simulink model "sampleModel1745"  (R2023a)
settings: Solver=VariableStepAuto  StartTime=0.0  StopTime=10.0  RelTol=1e-3
libraries: hdlsllib x3, simulink x2
settings Model: Creator=user1  LastModifiedBy=user1

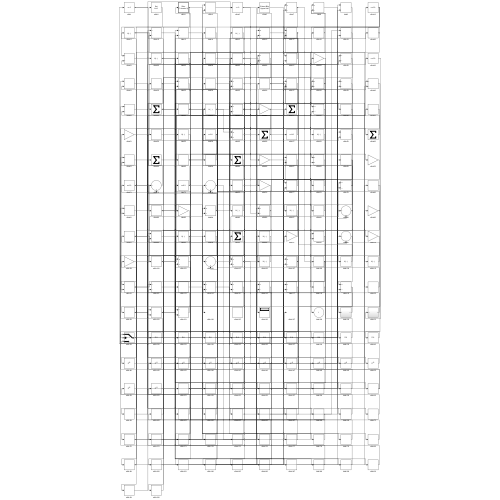
[thumbnail: Simulink's stored preview of the top-level diagram]
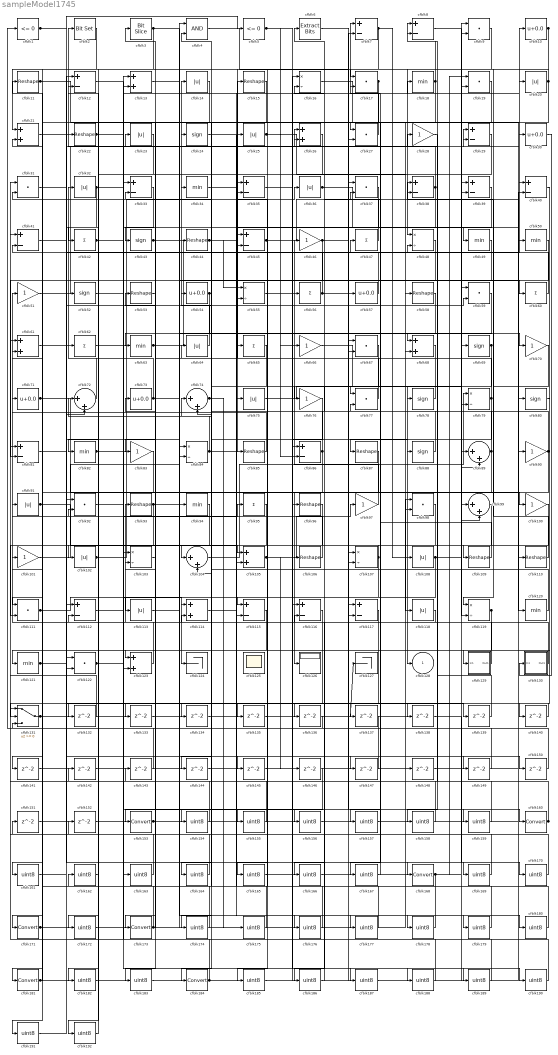
== system sampleModel1745 ==
  cfblk1 : hdlsllib/Logic and Bit Operations/Compare To Zero  relop=<=  OutDataTypeStr=boolean
  cfblk{10,30,54,57,71,73} (6 alike) : Bias  Bias=0.0  SaturateOnIntegerOverflow=off
  cfblk{28,46,51,66,70,76,83,90,97,100..101} (11 alike) : Gain
  cfblk{14,20,23,25,32,36,64,75,91,102,108,113,118} (13 alike) : Abs  SaturateOnIntegerOverflow=off
  cfblk{16,48,55,79,84,103,107,119} (8 alike) : Product  Inputs=*/  RndMeth=Zero  SaturateOnIntegerOverflow=on
  cfblk{72,74,89,99,104} (5 alike) : Sum  Inputs=|++
  cfblk{13,21,26,61,68,105,114,123} (8 alike) : Sum
  cfblk{11,15,22,44,53,58,85,87,93,96,106,109..110} (13 alike) : Reshape
  cfblk{9,17,19,27,31,37,59,67,77,92,98,111,122} (13 alike) : DotProduct  OutDataTypeStr=Inherit: Inherit via internal rule
  cfblk{7..8,12,29,33,35,38..41,45,81,86,112,115..117} (17 alike) : Sum  Inputs=+-
  cfblk{18,34,49..50,63,82,94,120..121} (9 alike) : MinMax
  cfblk124 : Terminator
  cfblk125 : Scope
      settings: Floating=on
  cfblk126 : Display
  cfblk127 : Terminator
  cfblk129 : Subsystem
      settings: LibrarySourceBlock=|
      | hdlsllib/Ports &
      | Subsystems/Subsystem
  cfblk130 : Subsystem
      settings: LibrarySourceBlock=|
      | hdlsllib/Ports &
      | Subsystems/Subsystem
  cfblk131 : Switch  SaturateOnIntegerOverflow=off  InputSameDT=off
  cfblk{132..152} (21 alike) : Delay  SampleTime=1
  cfblk{153,160,168,171,173,181,184} (7 alike) : DataTypeConversion  SaturateOnIntegerOverflow=off  RndMeth=Floor
  cfblk{154..159,161..167,169..170,172,174..180,182..183,185..192} (33 alike) : DataTypeConversion  OutDataTypeStr=uint8  SaturateOnIntegerOverflow=off  RndMeth=Floor
  cfblk2 : simulink/Logic and Bit Operations/Bit Set  iBit=0
      settings: LibrarySourceBlock=|
      | hdlsllib/Logic and Bit
      | Operations/Bit Set
  cfblk{24,43,52,69,78,80,88} (7 alike) : Signum
  cfblk3 : hdlsllib/Logic and Bit Operations/Bit Slice  lidx=7  ridx=0
  cfblk4 : Logic  AllPortsSameDT=off  OutDataTypeStr=boolean
  cfblk{42,47,56,60,62,65,95} (7 alike) : Sum  Inputs=+
  cfblk5 : hdlsllib/Logic and Bit Operations/Compare To Zero  relop=<=  OutDataTypeStr=boolean
  cfblk6 : simulink/Logic and Bit Operations/Extract Bits  bitsToExtract=Upper half  numBits=8  bitIdxRange=[0 7]  outScalingMode=Preserve fixed-point scaling
      settings: LibrarySourceBlock=|
      | hdlsllib/Logic and Bit
      | Operations/Extract Bits
  cfblk128 : Outport  VectorParamsAs1DForOutWhenUnconnected=off
  wires:
  cfblk123/1 -> cfblk51/1
  cfblk9/1 -> cfblk85/1
  cfblk68/1 -> cfblk128/1
  cfblk51/1 -> cfblk29/1
  cfblk117/1 -> cfblk181/1
  cfblk104/1 -> cfblk79/1
  cfblk82/1 -> cfblk36/1, cfblk25/1
  cfblk33/1 -> cfblk43/1
  cfblk111/1 -> cfblk124/1, cfblk26/1
  cfblk47/1 -> cfblk6/1
  cfblk85/1 -> cfblk71/1
  cfblk77/1 -> cfblk15/1
  cfblk120/1 -> cfblk91/1
  cfblk103/1 -> cfblk173/1
  cfblk45/1 -> cfblk10/1, cfblk189/1
  cfblk102/1 -> cfblk47/1, cfblk95/1
  cfblk19/1 -> cfblk27/1
  cfblk86/1 -> cfblk126/1, cfblk33/2
  cfblk97/1 -> cfblk46/1
  cfblk69/1 -> cfblk77/1, cfblk104/2, cfblk166/1
  cfblk7/1 -> cfblk65/1, cfblk108/1
  cfblk72/1 -> cfblk32/1
  cfblk10/1 -> cfblk48/1, cfblk42/1, cfblk109/1
  cfblk94/1 -> cfblk171/1
  cfblk71/1 -> cfblk100/1, cfblk138/1
  cfblk63/1 -> cfblk68/1, cfblk26/2
  cfblk38/1 -> cfblk2/1, cfblk55/2
  cfblk121/1 -> cfblk101/1, cfblk59/2, cfblk147/1
  cfblk48/1 -> cfblk114/1
  cfblk116/1 -> cfblk184/1
  cfblk40/1 -> cfblk129/1(In1)
  cfblk17/1 -> cfblk133/1, cfblk134/1
  cfblk4/1 -> cfblk107/1
  cfblk67/1 -> cfblk105/1
  cfblk57/1 -> cfblk23/1
  cfblk30/1 -> cfblk130/1(In1)
  cfblk92/1 -> cfblk160/1
  cfblk131/1 -> cfblk127/1, cfblk89/2
  cfblk66/1 -> cfblk79/2
  cfblk25/1 -> cfblk118/1, cfblk86/2
  cfblk73/1 -> cfblk52/1, cfblk180/1
  cfblk23/1 -> cfblk82/1
  cfblk1/1 -> cfblk5/1, cfblk72/2
  cfblk62/1 -> cfblk40/1
  cfblk20/1 -> cfblk98/2, cfblk17/1
  cfblk75/1 -> cfblk78/1
  cfblk106/1 -> cfblk64/1
  cfblk64/1 -> cfblk14/1
  cfblk26/1 -> cfblk115/1
  cfblk59/1 -> cfblk83/1
  cfblk55/1 -> cfblk56/1
  cfblk95/1 -> cfblk115/2
  cfblk27/1 -> cfblk7/1
  cfblk70/1 -> cfblk119/1
  cfblk8/1 -> cfblk99/2
  cfblk129/1(Out1) -> cfblk93/1
  cfblk13/1 -> cfblk70/1
  cfblk119/1 -> cfblk141/1, cfblk157/1
  cfblk14/1 -> cfblk111/1
  cfblk93/1 -> cfblk179/1, cfblk192/1
  cfblk101/1 -> cfblk4/1
  cfblk42/1 -> cfblk49/1, cfblk48/2
  cfblk107/1 -> cfblk104/1, cfblk185/1
  cfblk88/1 -> cfblk31/2
  cfblk54/1 -> cfblk113/1, cfblk24/1
  cfblk90/1 -> cfblk16/2, cfblk102/1
  cfblk18/1 -> cfblk8/1, cfblk87/1
  cfblk105/1 -> cfblk97/1, cfblk146/1
  cfblk109/1 -> cfblk77/2
  cfblk58/1 -> cfblk68/2
  cfblk32/1 -> cfblk122/2, cfblk154/1
  cfblk65/1 -> cfblk74/2
  cfblk56/1 -> cfblk45/2, cfblk150/1
  cfblk78/1 -> cfblk76/1
  cfblk89/1 -> cfblk4/2, cfblk121/1
  cfblk43/1 -> cfblk75/1, cfblk177/1
  cfblk108/1 -> cfblk69/1, cfblk123/2, cfblk186/1
  cfblk115/1 -> cfblk123/1
  cfblk81/1 -> cfblk62/1
  cfblk110/1 -> cfblk38/1
  cfblk91/1 -> cfblk105/2, cfblk50/1
  cfblk5/1 -> cfblk88/1, cfblk66/1
  cfblk61/1 -> cfblk84/2
  cfblk21/1 -> cfblk22/1
  cfblk130/1(Out1) -> cfblk61/2
  cfblk16/1 -> cfblk110/1
  cfblk36/1 -> cfblk119/2, cfblk120/1
  cfblk98/1 -> cfblk111/2
  cfblk15/1 -> cfblk63/1
  cfblk44/1 -> cfblk30/1, cfblk55/1
  cfblk6/1 -> cfblk57/1
  cfblk79/1 -> cfblk54/1, cfblk3/1, cfblk167/1
  cfblk74/1 -> cfblk44/1, cfblk175/1
  cfblk3/1 -> cfblk21/1, cfblk60/1
  cfblk53/1 -> cfblk153/1
  cfblk122/1 -> cfblk18/1, cfblk29/2
  cfblk96/1 -> cfblk106/1
  cfblk11/1 -> cfblk58/1, cfblk145/1
  cfblk46/1 -> cfblk159/1, cfblk174/1
  cfblk50/1 -> cfblk81/2
  cfblk60/1 -> cfblk21/2
  cfblk22/1 -> cfblk139/1, cfblk188/1
  cfblk41/1 -> cfblk168/1
  cfblk52/1 -> cfblk13/2
  cfblk84/1 -> cfblk20/1, cfblk72/1
  cfblk118/1 -> cfblk114/2
  cfblk29/1 -> cfblk132/1
  cfblk132/1 -> cfblk61/1
  cfblk133/1 -> cfblk84/1
  cfblk134/1 -> cfblk19/2
  cfblk113/1 -> cfblk135/1
  cfblk135/1 -> cfblk89/1
  cfblk24/1 -> cfblk136/1
  cfblk136/1 -> cfblk1/1
  cfblk100/1 -> cfblk137/1
  cfblk137/1 -> cfblk131/3
  cfblk139/1 -> cfblk38/2
  cfblk80/1 -> cfblk140/1
  cfblk140/1 -> cfblk131/2
  cfblk141/1 -> cfblk40/2
  cfblk142/1 -> cfblk7/2
  cfblk143/1 -> cfblk31/1
  cfblk76/1 -> cfblk144/1
  cfblk144/1 -> cfblk99/1
  cfblk145/1 -> cfblk67/1
  cfblk147/1 -> cfblk74/1
  cfblk148/1 -> cfblk59/1
  cfblk114/1 -> cfblk149/1
  cfblk149/1 -> cfblk45/1
  cfblk150/1 -> cfblk8/2
  cfblk151/1 -> cfblk27/2
  cfblk153/1 -> cfblk107/2, cfblk90/1, cfblk156/1
  cfblk154/1 -> cfblk53/1
  cfblk39/1 -> cfblk155/1
  cfblk155/1 -> cfblk142/1
  cfblk156/1 -> cfblk39/1
  cfblk157/1 -> cfblk39/2
  cfblk28/1 -> cfblk158/1
  cfblk158/1 -> cfblk98/1
  cfblk159/1 -> cfblk28/1
  cfblk160/1 -> cfblk17/2, cfblk81/1
  cfblk2/1 -> cfblk161/1
  cfblk161/1 -> cfblk92/1
  cfblk162/1 -> cfblk92/2
  cfblk152/1 -> cfblk163/1
  cfblk163/1 -> cfblk122/1
  cfblk87/1 -> cfblk164/1
  cfblk164/1 -> cfblk152/1
  cfblk37/1 -> cfblk165/1
  cfblk165/1 -> cfblk9/1
  cfblk166/1 -> cfblk37/1
  cfblk167/1 -> cfblk37/2
  cfblk168/1 -> cfblk162/1, cfblk19/1
  cfblk31/1 -> cfblk169/1
  cfblk169/1 -> cfblk41/1
  cfblk138/1 -> cfblk170/1
  cfblk170/1 -> cfblk41/2
  cfblk171/1 -> cfblk148/1, cfblk96/1
  cfblk83/1 -> cfblk172/1
  cfblk172/1 -> cfblk94/1
  cfblk173/1 -> cfblk143/1, cfblk86/1, cfblk33/1
  cfblk174/1 -> cfblk103/1
  cfblk175/1 -> cfblk103/2
  cfblk34/1 -> cfblk176/1
  cfblk176/1 -> cfblk73/1
  cfblk177/1 -> cfblk34/1
  cfblk35/1 -> cfblk178/1
  cfblk178/1 -> cfblk11/1
  cfblk179/1 -> cfblk35/1
  cfblk180/1 -> cfblk35/2
  cfblk181/1 -> cfblk151/1, cfblk16/1
  cfblk99/1 -> cfblk182/1
  cfblk182/1 -> cfblk117/1
  cfblk146/1 -> cfblk183/1
  cfblk183/1 -> cfblk117/2
  cfblk184/1 -> cfblk9/2, cfblk67/2, cfblk13/1
  cfblk185/1 -> cfblk116/1
  cfblk186/1 -> cfblk116/2
  cfblk12/1 -> cfblk187/1
  cfblk187/1 -> cfblk80/1
  cfblk188/1 -> cfblk12/1
  cfblk189/1 -> cfblk12/2
  cfblk112/1 -> cfblk190/1
  cfblk190/1 -> cfblk131/1
  cfblk49/1 -> cfblk191/1
  cfblk191/1 -> cfblk112/1
  cfblk192/1 -> cfblk112/2

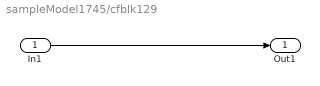
== system sampleModel1745/cfblk129 ==
  In1 : Inport
  Out1 : Outport
  wires:
  In1/1 -> Out1/1

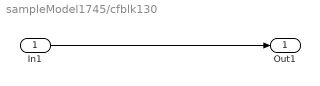
== system sampleModel1745/cfblk130 ==
  In1 : Inport
  Out1 : Outport
  wires:
  In1/1 -> Out1/1
